simulink model "LazoCerrado"  (R2023a)
settings: Solver=ode15s  StartTime=0.0  StopTime=30  MaxStep=1E-3  RelTol=1e-3
libraries: slpidlib x1
settings Model: Creator=jesus  LastModifiedBy=jesus
settings DataIOCC: ReturnWorkspaceOutputs=off  TimeSaveName=t
settings DebuggingCC: AlgebraicLoopMsg=none  ArtificialAlgebraicLoopMsg=none  MaxConsecutiveZCsMsg=none  ModelReferenceExtraNoncontSigs=none  OperatingPointInterfaceChecksumMismatchMsg=none

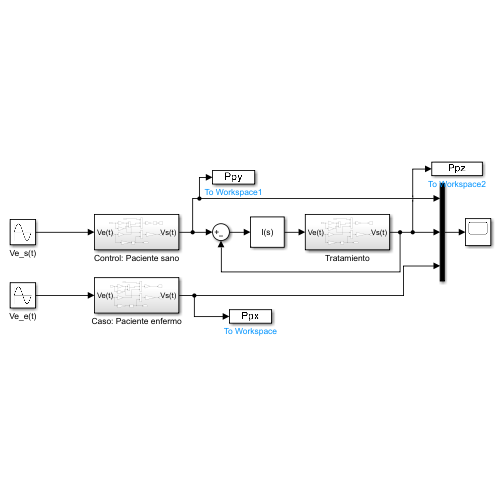
[thumbnail: Simulink's stored preview of the top-level diagram]
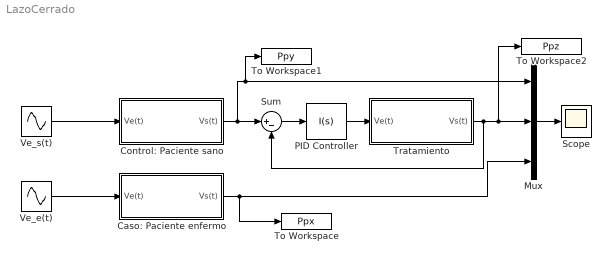
== system LazoCerrado ==
  Caso: Paciente enfermo : Subsystem
  Control: Paciente sano : Subsystem
  Mux : Mux  Inputs=3
  PID Controller : slpidlib/PID Controller  Controller=I  Form=Parallel  TimeDomain=Continuous-time  UseExternalTs=off  SampleTime=-1  IntegratorMethod=Forward Euler  FilterMethod=Forward Euler  ControllerParametersSource=internal  P=0  I=1929.48273797327  UseKiTs=off  D=0  N=1  UseFilter=on  TunerSelectOption=Transfer Function Based (PID Tuner App)  InitialConditionSource=internal  InitialConditionForIntegrator=0  InitialConditionForFilter=0  DifferentiatorICPrevScaledInput=0  ExternalReset=none  TrackingMode=off  Kt=1  LimitOutput=off  SatLimitsSource=internal  UpperSaturationLimit=inf  LowerSaturationLimit=-inf  LinearizeAsGain=on  AntiWindupMode=none  Kb=1  LimitIntegrator=off  UpperIntegratorSaturationLimit=inf  LowerIntegratorSaturationLimit=-inf  POutMin=[]  POutMax=[]  IOutMin=[]  IOutMax=[]  DOutMin=[]  DOutMax=[]  NOutMin=[]  NOutMax=[]  SumOutMin=[]  SumOutMax=[]  SaturationOutMin=[]  SaturationOutMax=[]  PParamMin=[]  PParamMax=[]  IParamMin=[]  IParamMax=[]  DParamMin=[]  DParamMax=[]  NParamMin=[]  NParamMax=[]  KbParamMin=[]  KbParamMax=[]  KtParamMin=[]  KtParamMax=[]  KbOutMin=[]  KbOutMax=[]  KtOutMin=[]  KtOutMax=[]  IntegratorOutMin=[]  IntegratorOutMax=[]  FilterOutMin=[]  FilterOutMax=[]  SumI1OutMin=[]  SumI1OutMax=[]  SumI2OutMin=[]  SumI2OutMax=[]  SumI3OutMin=[]  SumI3OutMax=[]  SumI4OutMin=[]  SumI4OutMax=[]  SumDOutMin=[]  SumDOutMax=[]  DifferentiatorOutMin=[]  DifferentiatorOutMax=[]  FilterDiffOutCoefMin=[]  FilterDiffOutCoefMax=[]  ReciprocalOutMin=[]  ReciprocalOutMax=[]  SumDenOutMin=[]  SumDenOutMax=[]  SumNumOutMin=[]  SumNumOutMax=[]  DivideOutMin=[]  DivideOutMax=[]  UdiffTsProdOutMin=[]  UdiffTsProdOutMax=[]  NTsProdOutMin=[]  NTsProdOutMax=[]  UintegralTsProdOutMin=[]  UintegralTsProdOutMax=[]  UngainTsProdOutMin=[]  UngainTsProdOutMax=[]  ClampingZeroOutDataTypeStr=Inherit: Inherit via back propagation  ClampingZeroOutMin=[]  ClampingZeroOutMax=[]  FilterDenConstantOutDataTypeStr=Inherit: Inherit via back propagation  FilterDenConstantOutMin=[]  FilterDenConstantOutMax=[]  PCopyOutDataTypeStr=Inherit: Inherit via back propagation  PCopyOutMin=[]  PCopyOutMax=[]  NCopyOutDataTypeStr=Inherit: Inherit via back propagation  NCopyOutMin=[]  NCopyOutMax=[]  IntegratorContinuousStateAttributes=''  IntegratorStateMustResolveToSignalObject=off  IntegratorRTWStateStorageClass=Auto  FilterContinuousStateAttributes=''  FilterStateMustResolveToSignalObject=off  FilterRTWStateStorageClass=Auto  ParallelPVariant=Disabled  IdealPVariant=Disabled  IVariant=InternalParameters  DVariant=Disabled  IntegratorVariant=Continuous  SatVariant=Disabled  AWVariant=Passthrough  PCopyVariant=Disabled  TRVariant=Disabled  FdbkBlocksVariant=Forward  IdealPFdbkVariant=Disabled  SatFdbkVariant=Disabled  DerivativeFilterVariant=Disabled  NVariant=Disabled  NCopyVariant=Disabled_SignalSpec  FilterICVariant=Disabled  IntegratorICVariant=InternalICs  ExternalResetVariant=Disabled  TRSumVariant=Passthrough  SumFdbkVariant=Disabled  SumVariant=Passthrough_I  TsampFilterVariant=InternalTs  TsampNgainVariant=Passthrough  TsampIntegralVariant=Disabled_SignalSpec  ExternalSaturationOutDataTypeStr=Inherit: Same as second input
  Scope : Scope
  Sum : Sum  Inputs=|+-
  To Workspace : ToWorkspace  VariableName=Ppx  SampleTime=-1
  To Workspace1 : ToWorkspace  VariableName=Ppy  SampleTime=-1
  To Workspace2 : ToWorkspace  VariableName=Ppz  SampleTime=-1
  Tratamiento : Subsystem
  Ve_e(t) : Sin  Amplitude=0.4  Frequency=2*pi  SampleTime=0
  Ve_s(t) : Sin  Frequency=2*pi  SampleTime=0
  wires:
  PID Controller/1 -> Tratamiento/1(Ve(t))
  Sum/1 -> PID Controller/1
  Tratamiento/1(Vs(t)) -> To Workspace2/1, Mux/2, Sum/2
  Control: Paciente sano/1(Vs(t)) -> To Workspace1/1, Mux/1, Sum/1
  Caso: Paciente enfermo/1(Vs(t)) -> To Workspace/1, Mux/3
  Mux/1 -> Scope/1
  Ve_s(t)/1 -> Control: Paciente sano/1(Ve(t))
  Ve_e(t)/1 -> Caso: Paciente enfermo/1(Ve(t))

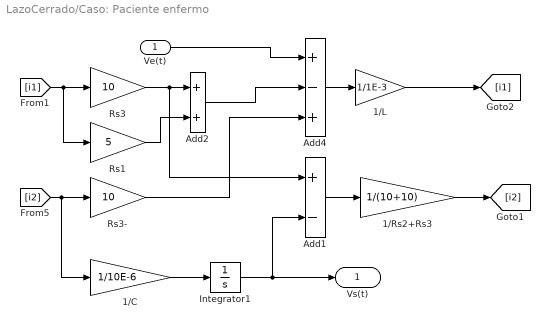
== system LazoCerrado/Caso: Paciente enfermo ==
  Ve(t) : Inport
  1/C : Gain  Gain=1/10E-6
  1/L : Gain  Gain=1/1E-3
  1/Rs2+Rs3 : Gain  Gain=1/(10+10)
  Add1 : Sum  Inputs=+-
  Add2 : Sum
  Add4 : Sum  Inputs=+-+
  Integrator1 : Integrator
  Rs1 : Gain  Gain=5
  Rs3 : Gain  Gain=10
  Rs3- : Gain  Gain=10
  Vs(t) : Outport
  wires:
  Add1/1 -> 1/Rs2+Rs3/1
  Rs1/1 -> Add2/2
  [i2] -> 1/C/1, Rs3-/1
  [i1] -> Rs1/1, Rs3/1
  1/Rs2+Rs3/1 -> [i2]
  Ve(t)/1 -> Add4/1
  Rs3/1 -> Add2/1, Add1/1
  Add4/1 -> 1/L/1
  1/C/1 -> Integrator1/1
  Add2/1 -> Add4/2
  Rs3-/1 -> Add4/3
  Integrator1/1 -> Vs(t)/1, Add1/2
  1/L/1 -> [i1]

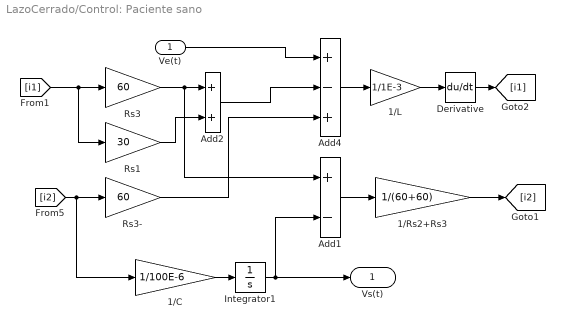
== system LazoCerrado/Control: Paciente sano ==
  Ve(t) : Inport
  1/C : Gain  Gain=1/100E-6
  1/L : Gain  Gain=1/1E-3
  1/Rs2+Rs3 : Gain  Gain=1/(60+60)
  Add1 : Sum  Inputs=+-
  Add2 : Sum
  Add4 : Sum  Inputs=+-+
  Derivative : Derivative
  Integrator1 : Integrator
  Rs1 : Gain  Gain=30
  Rs3 : Gain  Gain=60
  Rs3- : Gain  Gain=60
  Vs(t) : Outport
  wires:
  Ve(t)/1 -> Add4/1
  Add4/1 -> 1/L/1
  [i1] -> Rs1/1, Rs3/1
  [i2] -> 1/C/1, Rs3-/1
  Rs3/1 -> Add2/1, Add1/1
  Rs1/1 -> Add2/2
  Add2/1 -> Add4/2
  Rs3-/1 -> Add4/3
  1/L/1 -> Derivative/1
  1/Rs2+Rs3/1 -> [i2]
  1/C/1 -> Integrator1/1
  Integrator1/1 -> Add1/2, Vs(t)/1
  Add1/1 -> 1/Rs2+Rs3/1
  Derivative/1 -> [i1]

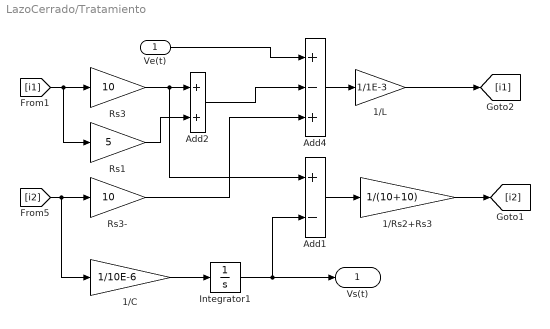
== system LazoCerrado/Tratamiento ==
  Ve(t) : Inport
  1/C : Gain  Gain=1/10E-6
  1/L : Gain  Gain=1/1E-3
  1/Rs2+Rs3 : Gain  Gain=1/(10+10)
  Add1 : Sum  Inputs=+-
  Add2 : Sum
  Add4 : Sum  Inputs=+-+
  Integrator1 : Integrator
  Rs1 : Gain  Gain=5
  Rs3 : Gain  Gain=10
  Rs3- : Gain  Gain=10
  Vs(t) : Outport
  wires:
  Add1/1 -> 1/Rs2+Rs3/1
  Rs1/1 -> Add2/2
  [i2] -> 1/C/1, Rs3-/1
  [i1] -> Rs1/1, Rs3/1
  1/Rs2+Rs3/1 -> [i2]
  Ve(t)/1 -> Add4/1
  Rs3/1 -> Add2/1, Add1/1
  Add4/1 -> 1/L/1
  1/C/1 -> Integrator1/1
  Add2/1 -> Add4/2
  Rs3-/1 -> Add4/3
  Integrator1/1 -> Vs(t)/1, Add1/2
  1/L/1 -> [i1]
